simulink model "ClosedLoopSys"  (R2023b)
settings: Solver=VariableStepAuto  StartTime=0.00  StopTime=60.00  FixedStep=T  RelTol=1e-5  EnableMultiTasking=on
values from neighbouring files (symbols this model uses):
  amp_sat_l = 0    [heli_new.m]
  amp_sat_u = 12    [heli_new.m]
  b = fir1(200, 0.004)    [heli_new.m]
  Cr = [1,0,0,0,0,0 ... (first row only)    [heli_new.m]
  DAC_lim_l = 0    [heli_new.m]
  DAC_lim_u = 10    [heli_new.m]
  e_lim_l = min(ElevAxisData.Var1)*pi/180    [heli_new.m]
  Fss_ab = ThrustMeas.Var2    [heli_new.m]
  g = 9.81    [heli_new.m]
  Je = 2*m1*(l1^2)+m2*(l3^2)    (= 0.0023885)    [heli_new.m]
  Jp = 2*m1*(l2^2)    (= 0.0004949)    [heli_new.m]
  Jt = Je    (= 0.0023885)    [heli_new.m]
  K = Kaug(:,1:6)    [heli_new.m]
  k_a = 1.2    [heli_new.m]
  k_d = 0.0005    [heli_new.m]
  k_s = 0.0015    [heli_new.m]
  ki = -Kaug(:,7:8)    [heli_new.m]
  l1 = 0.110    (= 0.11)    [heli_new.m]
  l2 = 0.070    (= 0.07)    [heli_new.m]
  l3 = 0.108    [heli_new.m]
  m1 = 0.0505    [heli_new.m]
  m2 = 0.100    (= 0.1)    [heli_new.m]
  T = 0.02    [heli_new.m]
  tau = 0.6    [heli_new.m]
  U_e = 3.8    [heli_new.m]
  V_ab = ThrustMeas.Var1    [heli_new.m]
undefined symbols (not defined in the file or in its folder): DiscIntNeverNeededParam, kdfilt
settings Model: Creator=bjones  LastModifiedBy=GCRAFT
settings SolverCC: AlgebraicLoopSolver=TrustRegion
settings DataIOCC: SaveFormat=Array  SignalLoggingSaveFormat=ModelDataLogs  ReturnWorkspaceOutputs=off
settings OptimizationCC: BlockReduction=off  BooleanDataType=off  ExpressionDepthLimit=2147483647  LifeSpan=inf
settings DebuggingCC: SaveWithParameterizedLinksMsg=none  UnderspecifiedInitializationDetection=Classic  MergeDetectMultiDrivingBlocksExec=none  SignalResolutionControl=TryResolveAllWithWarning  MultiTaskDSMMsg=warning  MultiTaskCondExecSysMsg=none  FcnCallInpInsideContextMsg=warning  UnconnectedInputMsg=warning  UnconnectedOutputMsg=warning  UnconnectedLineMsg=warning  StateNameClashWarn=warning  SFUnexpectedBacktrackingDiag=warning  SFNoUnconditionalDefaultTransitionDiag=warning  SFExecutionAtInitializationDiag=none  ArithmeticOperatorsInVariantConditions=warning
settings HardwareCC: ProdBitPerPointer=32  ProdBitPerSizeT=32  ProdBitPerPtrDiffT=32  ProdLargestAtomicFloat=None  ProdIntDivRoundTo=Undefined  ProdEndianess=Unspecified  ProdWordSize=32  ProdHWDeviceType=32-bit Generic  TargetUnknown=on
settings ModelReferenceCC: EnableRefExpFcnMdlSchedulingChecks=on  PropagateSignalLabelsOutOfModel=off
settings SFSimCC: SimUseLocalCustomCode=off  CustomCodeUndefinedFunction=UseInterfaceOnly
settings RTWCC: RTWUseLocalCustomCode=off
settings CodeAppCC: StateflowObjectComments=on
settings GRTTargetCC: TargetLangStandard=C89/C90 (ANSI)  CombineOutputUpdateFcns=off  GRTInterface=on
settings ConfigComp: CovMetricSettings=dw  CovSaveCumulativeToWorkspaceVar=on  CovSaveSingleToWorkspaceVar=on  CovExternalEMLEnable=off  CovSFcnEnable=off

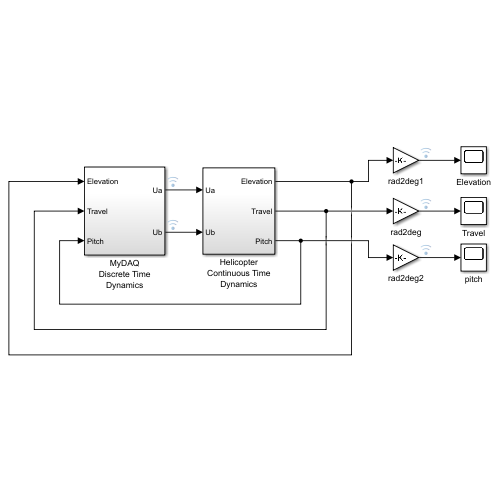
[thumbnail: Simulink's stored preview of the top-level diagram]
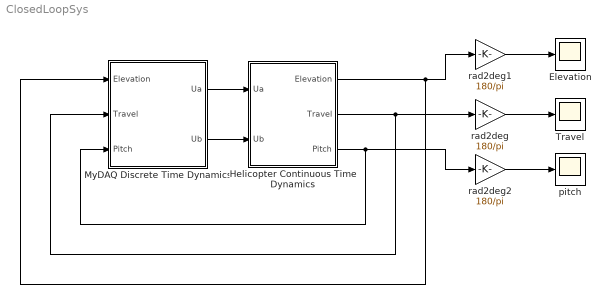
== system ClosedLoopSys ==
  Elevation : Scope
  Helicopter Continuous Time Dynamics : Subsystem
  MyDAQ Discrete Time Dynamics : Subsystem
  Travel : Scope
  pitch : Scope
  rad2deg : Gain  Gain=180/pi  SaturateOnIntegerOverflow=on  OutDataTypeStr=Inherit: Same as input  ParamDataTypeStr=Inherit: Same as input
  rad2deg1 : Gain  Gain=180/pi  SaturateOnIntegerOverflow=on  OutDataTypeStr=Inherit: Same as input  ParamDataTypeStr=Inherit: Same as input
  rad2deg2 : Gain  Gain=180/pi  SaturateOnIntegerOverflow=on  OutDataTypeStr=Inherit: Same as input  ParamDataTypeStr=Inherit: Same as input
  wires:
  rad2deg/1 -> Travel/1
  rad2deg1/1 -> Elevation/1
  Helicopter Continuous Time Dynamics/2(Travel) -> MyDAQ Discrete Time Dynamics/2(Travel), rad2deg/1
  Helicopter Continuous Time Dynamics/1(Elevation) -> rad2deg1/1, MyDAQ Discrete Time Dynamics/1(Elevation)
  rad2deg2/1 -> pitch/1
  Helicopter Continuous Time Dynamics/3(Pitch) -> rad2deg2/1, MyDAQ Discrete Time Dynamics/3(Pitch)
  MyDAQ Discrete Time Dynamics/1(Ua) -> Helicopter Continuous Time Dynamics/1(Ua)
  MyDAQ Discrete Time Dynamics/2(Ub) -> Helicopter Continuous Time Dynamics/2(Ub)

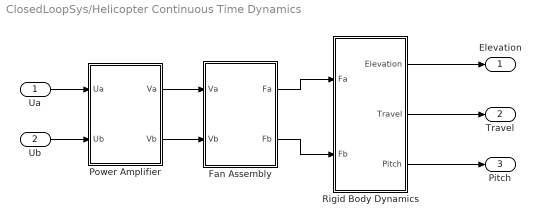
== system ClosedLoopSys/Helicopter Continuous Time Dynamics ==
  Ua : Inport
  Ub : Inport  Port=2
  Fan Assembly : Subsystem
  Power Amplifier : Subsystem
  Rigid Body Dynamics : Subsystem
  Elevation : Outport
  Travel : Outport  Port=2
  Pitch : Outport  Port=3
  wires:
  Power Amplifier/1(Va) -> Fan Assembly/1(Va)
  Power Amplifier/2(Vb) -> Fan Assembly/2(Vb)
  Rigid Body Dynamics/1(Elevation) -> Elevation/1
  Rigid Body Dynamics/3(Pitch) -> Pitch/1
  Fan Assembly/2(Fb) -> Rigid Body Dynamics/2(Fb)
  Ua/1 -> Power Amplifier/1(Ua)
  Ub/1 -> Power Amplifier/2(Ub)
  Rigid Body Dynamics/2(Travel) -> Travel/1
  Fan Assembly/1(Fa) -> Rigid Body Dynamics/1(Fa)

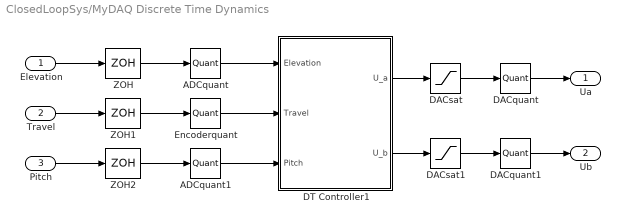
== system ClosedLoopSys/MyDAQ Discrete Time Dynamics ==
  Elevation : Inport
  Travel : Inport  Port=2
  Pitch : Inport  Port=3
  ADCquant : Quantizer  QuantizationInterval=ADC_Vres  SampleTime=T
  ADCquant1 : Quantizer  QuantizationInterval=ADC_Vres  SampleTime=T
  DACquant : Quantizer  QuantizationInterval=DAC_Vres  SampleTime=T
  DACquant1 : Quantizer  QuantizationInterval=DAC_Vres  SampleTime=T
  DACsat : Saturate  UpperLimit=DAC_lim_u  LowerLimit=DAC_lim_l  SampleTime=T
  DACsat1 : Saturate  UpperLimit=DAC_lim_u  LowerLimit=DAC_lim_l  SampleTime=T
  DT Controller1 : Subsystem
  Encoderquant : Quantizer  QuantizationInterval=Encoder_res  SampleTime=T
  ZOH : ZeroOrderHold  SampleTime=T
  ZOH1 : ZeroOrderHold  SampleTime=T
  ZOH2 : ZeroOrderHold  SampleTime=T
  Ua : Outport
  Ub : Outport  Port=2
  wires:
  Elevation/1 -> ZOH/1
  Travel/1 -> ZOH1/1
  DACquant/1 -> Ua/1
  DACquant1/1 -> Ub/1
  DT Controller1/1(U_a) -> DACsat/1
  DACsat/1 -> DACquant/1
  DT Controller1/2(U_b) -> DACsat1/1
  DACsat1/1 -> DACquant1/1
  ZOH1/1 -> Encoderquant/1
  ZOH/1 -> ADCquant/1
  Pitch/1 -> ZOH2/1
  ZOH2/1 -> ADCquant1/1
  ADCquant/1 -> DT Controller1/1(Elevation)
  ADCquant1/1 -> DT Controller1/3(Pitch)
  Encoderquant/1 -> DT Controller1/2(Travel)

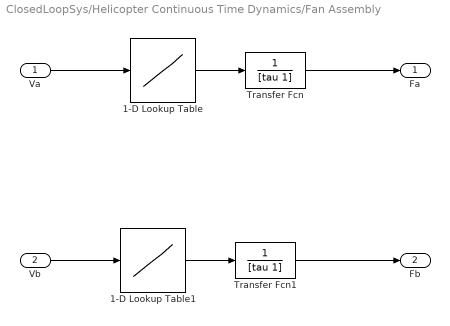
== system ClosedLoopSys/Helicopter Continuous Time Dynamics/Fan Assembly ==
  Va : Inport
  Vb : Inport  Port=2
  1-D Lookup Table : Lookup_n-D  NumberOfTableDimensions=1  LookupTableObject=ThrustMeas  BreakpointsForDimension1=V_ab  Table=Fss_ab  InternalRulePriority=Speed  RndMeth=Simplest
  1-D Lookup Table1 : Lookup_n-D  NumberOfTableDimensions=1  LookupTableObject=ThrustMeas  BreakpointsForDimension1=V_ab  Table=Fss_ab  InternalRulePriority=Speed  RndMeth=Simplest
  Transfer Fcn : TransferFcn  Denominator=[tau 1]
  Transfer Fcn1 : TransferFcn  Denominator=[tau 1]
  Fa : Outport
  Fb : Outport  Port=2
  wires:
  1-D Lookup Table/1 -> Transfer Fcn/1
  Transfer Fcn1/1 -> Fb/1
  1-D Lookup Table1/1 -> Transfer Fcn1/1
  Vb/1 -> 1-D Lookup Table1/1
  Va/1 -> 1-D Lookup Table/1
  Transfer Fcn/1 -> Fa/1

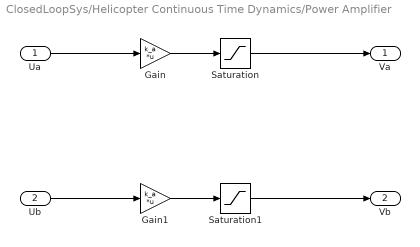
== system ClosedLoopSys/Helicopter Continuous Time Dynamics/Power Amplifier ==
  Ua : Inport
  Ub : Inport  Port=2
  Gain : Gain  Gain=k_a  Multiplication=Matrix(K*u)
  Gain1 : Gain  Gain=k_a  Multiplication=Matrix(K*u)
  Saturation : Saturate  UpperLimit=amp_sat_u  LowerLimit=amp_sat_l
  Saturation1 : Saturate  UpperLimit=amp_sat_u  LowerLimit=amp_sat_l
  Va : Outport
  Vb : Outport  Port=2
  wires:
  Gain/1 -> Saturation/1
  Gain1/1 -> Saturation1/1
  Saturation1/1 -> Vb/1
  Ub/1 -> Gain1/1
  Ua/1 -> Gain/1
  Saturation/1 -> Va/1

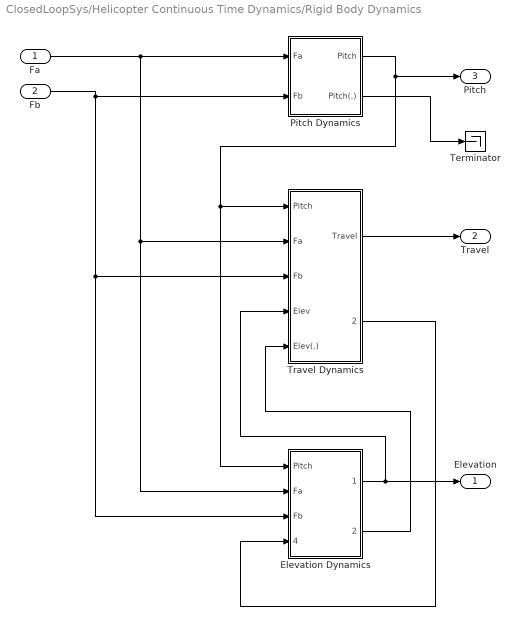
== system ClosedLoopSys/Helicopter Continuous Time Dynamics/Rigid Body Dynamics ==
  Fa : Inport
  Fb : Inport  Port=2
  Elevation Dynamics : Subsystem
  Pitch Dynamics : Subsystem
  Terminator : Terminator
  Travel Dynamics : Subsystem
  Elevation : Outport
  Travel : Outport  Port=2
  Pitch : Outport  Port=3
  wires:
  Fa/1 -> Pitch Dynamics/1(Fa), Travel Dynamics/2(Fa), Elevation Dynamics/2(Fa)
  Fb/1 -> Pitch Dynamics/2(Fb), Elevation Dynamics/3(Fb), Travel Dynamics/3(Fb)
  Travel Dynamics/1(Travel) -> Travel/1
  Elevation Dynamics/1(Elevation) -> Elevation/1, Travel Dynamics/4(Elev)
  Pitch Dynamics/1(Pitch) -> Travel Dynamics/1(Pitch), Elevation Dynamics/1(Pitch), Pitch/1
  Travel Dynamics/2(Travel(.)) -> Elevation Dynamics/4(Travel(.))
  Elevation Dynamics/2(Elevation(.)) -> Travel Dynamics/5(Elev(.))
  Pitch Dynamics/2("Pitch(.) ") -> Terminator/1

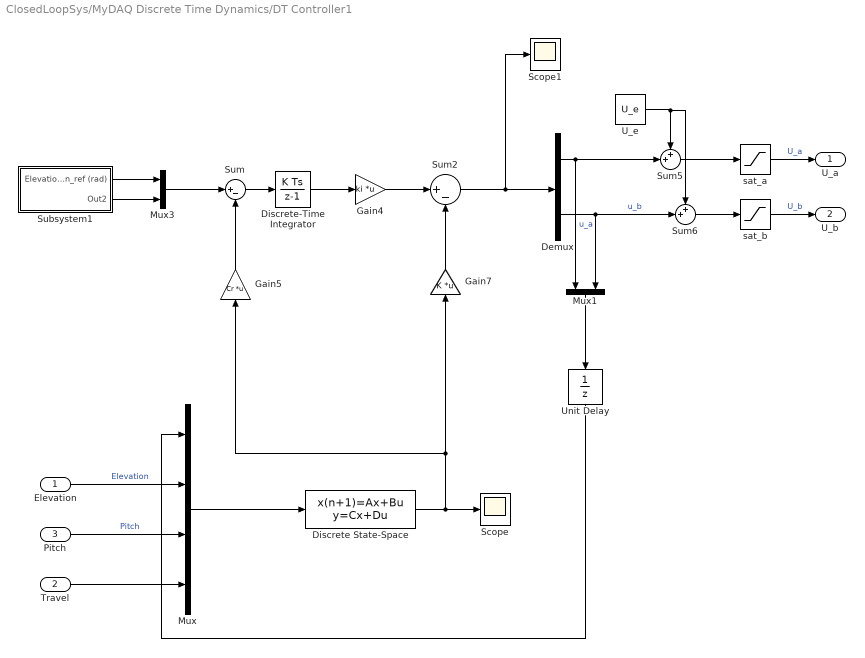
== system ClosedLoopSys/MyDAQ Discrete Time Dynamics/DT Controller1 ==
  Elevation : Inport
  Travel : Inport  Port=2
  Pitch : Inport  Port=3
  Demux : Demux  Outputs=2
  Discrete State-Space : DiscreteStateSpace  A=kdfilt.a  B=kdfilt.b  C=kdfilt.c(size(C,1)+1:end,:)  D=kdfilt.d(size(C,1)+1:end,:)  InitialCondition=[e_lim_l; 0; 0; 0; 0; 0]  SampleTime=T
  Discrete-Time Integrator : DiscreteIntegrator  SampleTime=T  ICPrevOutput=DiscIntNeverNeededParam  ICPrevScaledInput=DiscIntNeverNeededParam
  Gain4 : Gain  Gain=ki  Multiplication=Matrix(K*u)
  Gain5 : Gain  Gain=Cr  Multiplication=Matrix(K*u)
  Gain7 : Gain  Gain=K  Multiplication=Matrix(K*u)
  Mux : Mux
  Mux1 : Mux  Inputs=2
  Mux3 : Mux  Inputs=2
  Scope : Scope
  Scope1 : Scope
  Subsystem1 : Subsystem
  Sum : Sum  Inputs=|+-
  Sum2 : Sum  Inputs=|+-
  Sum5 : Sum  Inputs=++|
  Sum6 : Sum  Inputs=++|
  U_e : Constant  Value=U_e  SampleTime=T
  Unit Delay : UnitDelay  SampleTime=T  HasFrameUpgradeWarning=on
  sat_a : Saturate  UpperLimit=DAC_lim_u  LowerLimit=DAC_lim_l
  sat_b : Saturate  UpperLimit=DAC_lim_u  LowerLimit=DAC_lim_l
  U_a : Outport
  U_b : Outport  Port=2
  wires:
  U_e/1 -> Sum6/1, Sum5/1
  Sum5/1 -> sat_a/1
  Sum6/1 -> sat_b/1
  Demux/1 -> Sum5/2, Mux1/1  "u_a"
  Demux/2 -> Sum6/2, Mux1/2  "u_b"
  Elevation/1 -> Mux/2  "Elevation"
  Discrete-Time Integrator/1 -> Gain4/1
  Sum2/1 -> Scope1/1, Demux/1
  Gain4/1 -> Sum2/1
  Sum/1 -> Discrete-Time Integrator/1
  Pitch/1 -> Mux/3  "Pitch"
  Travel/1 -> Mux/4
  Mux/1 -> Discrete State-Space/1
  Mux1/1 -> Unit Delay/1
  Unit Delay/1 -> Mux/1
  Discrete State-Space/1 -> Scope/1, Gain5/1, Gain7/1
  Mux3/1 -> Sum/1
  Gain5/1 -> Sum/2
  Gain7/1 -> Sum2/2
  Subsystem1/1(Elevation_ref (rad)) -> Mux3/1
  Subsystem1/2(Out2) -> Mux3/2
  sat_a/1 -> U_a/1  "U_a"
  sat_b/1 -> U_b/1  "U_b"

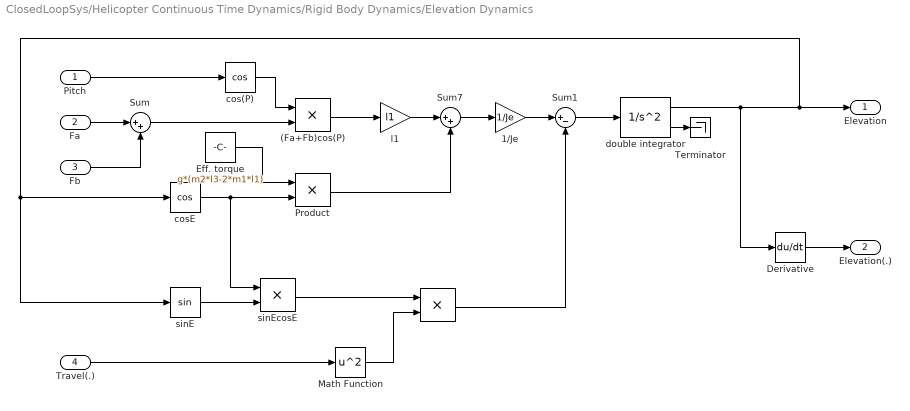
== system ClosedLoopSys/Helicopter Continuous Time Dynamics/Rigid Body Dynamics/Elevation Dynamics ==
  Pitch : Inport
  Fa : Inport  Port=2
  Fb : Inport  Port=3
  Travel(.) : Inport  Port=4
  " " : Product  InputSameDT=on  RndMeth=Zero  SaturateOnIntegerOverflow=on  OutDataTypeStr=Inherit: Same as first input
  (Fa+Fb)cos(P) : Product  InputSameDT=on  RndMeth=Zero  SaturateOnIntegerOverflow=on  OutDataTypeStr=Inherit: Same as first input
  1/Je : Gain  Gain=1/Je  SaturateOnIntegerOverflow=on  OutDataTypeStr=Inherit: Same as input  ParamDataTypeStr=Inherit: Same as input
  Derivative : Derivative
  Eff. torque : Constant  Value=g*(m2*l3-2*m1*l1)
  Math Function : Math  Operator=square  SignedPower=on
  Product : Product  InputSameDT=on  RndMeth=Zero  SaturateOnIntegerOverflow=on  OutDataTypeStr=Inherit: Same as first input
  Sum : Sum  Inputs=|++  InputSameDT=on  SaturateOnIntegerOverflow=on  OutDataTypeStr=Inherit: Same as first input
  Sum1 : Sum  Inputs=|+-  InputSameDT=on  SaturateOnIntegerOverflow=on  OutDataTypeStr=Inherit: Same as first input
  Sum7 : Sum  Inputs=|++  InputSameDT=on  SaturateOnIntegerOverflow=on  OutDataTypeStr=Inherit: Same as first input
  Terminator : Terminator
  cos(P) : Trigonometry  Operator=cos
  cosE : Trigonometry  Operator=cos
  double integrator : SecondOrderIntegrator  ICX=e_lim_l  LimitX=on  UpperLimitX=e_lim_u  LowerLimitX=e_lim_l  LimitDXDT=on  UpperLimitDXDT=2*pi  LowerLimitDXDT=-2*pi
  l1 : Gain  Gain=l1  SaturateOnIntegerOverflow=on  OutDataTypeStr=Inherit: Same as input  ParamDataTypeStr=Inherit: Same as input
  sinE : Trigonometry
  sinEcosE : Product  InputSameDT=on  RndMeth=Zero  SaturateOnIntegerOverflow=on  OutDataTypeStr=Inherit: Same as first input
  Elevation : Outport
  Elevation(.) : Outport  Port=2
  wires:
  double integrator/1 -> cosE/1, sinE/1, Elevation/1, Derivative/1
  Derivative/1 -> Elevation(.)/1
  double integrator/2 -> Terminator/1
  Fa/1 -> Sum/1
  Fb/1 -> Sum/2
  Sum/1 -> (Fa+Fb)cos(P)/2
  Pitch/1 -> cos(P)/1
  cos(P)/1 -> (Fa+Fb)cos(P)/1
  (Fa+Fb)cos(P)/1 -> l1/1
  l1/1 -> Sum7/1
  cosE/1 -> sinEcosE/1, Product/2
  Eff. torque/1 -> Product/1
  sinE/1 -> sinEcosE/2
  Product/1 -> Sum7/2
  Sum7/1 -> 1/Je/1
  1/Je/1 -> Sum1/1
  Travel(.)/1 -> Math Function/1
  Math Function/1 -> " "/2
  sinEcosE/1 -> " "/1
  " "/1 -> Sum1/2
  Sum1/1 -> double integrator/1

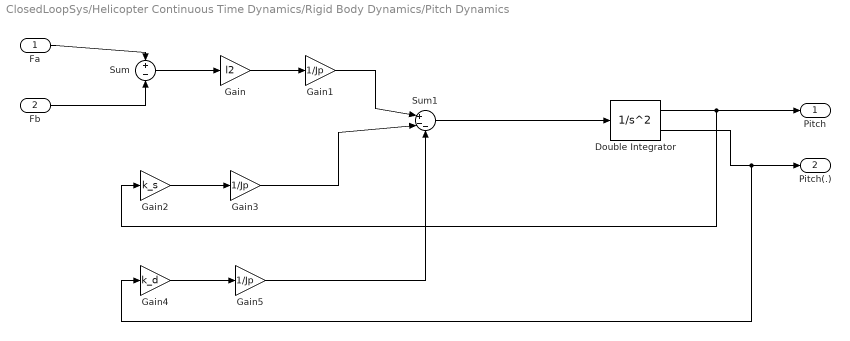
== system ClosedLoopSys/Helicopter Continuous Time Dynamics/Rigid Body Dynamics/Pitch Dynamics ==
  Fa : Inport
  Fb : Inport  Port=2
  Double Integrator : SecondOrderIntegrator  ICX=0  LimitX=on  UpperLimitX=p_lim_u  LowerLimitX=p_lim_l
  Gain : Gain  Gain=l2
  Gain1 : Gain  Gain=1/Jp
  Gain2 : Gain  Gain=k_s
  Gain3 : Gain  Gain=1/Jp
  Gain4 : Gain  Gain=k_d
  Gain5 : Gain  Gain=1/Jp
  Sum : Sum  Inputs=+-
  Sum1 : Sum  Inputs=|+--
  Pitch : Outport
  "Pitch(.) " : Outport  Port=2
  wires:
  Double Integrator/1 -> Gain2/1, Pitch/1
  Fa/1 -> Sum/1
  Fb/1 -> Sum/2
  Sum/1 -> Gain/1
  Gain/1 -> Gain1/1
  Gain1/1 -> Sum1/1
  Gain2/1 -> Gain3/1
  Gain3/1 -> Sum1/2
  Gain4/1 -> Gain5/1
  Gain5/1 -> Sum1/3
  Sum1/1 -> Double Integrator/1
  Double Integrator/2 -> Gain4/1, "Pitch(.) "/1

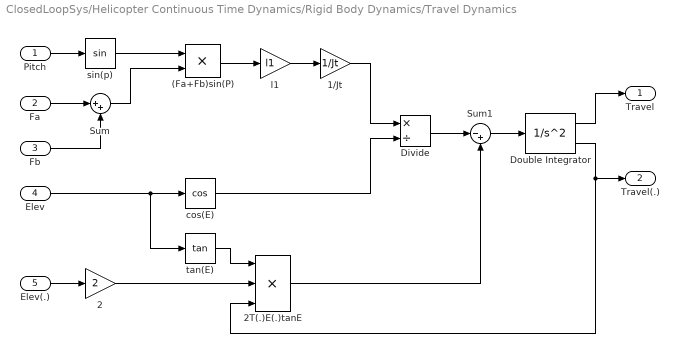
== system ClosedLoopSys/Helicopter Continuous Time Dynamics/Rigid Body Dynamics/Travel Dynamics ==
  Pitch : Inport
  Fa : Inport  Port=2
  Fb : Inport  Port=3
  Elev : Inport  Port=4
  Elev(.) : Inport  Port=5
  (Fa+Fb)sin(P) : Product  InputSameDT=on  RndMeth=Zero  SaturateOnIntegerOverflow=on  OutDataTypeStr=Inherit: Same as first input
  1/Jt : Gain  Gain=1/Jt  SaturateOnIntegerOverflow=on  OutDataTypeStr=Inherit: Same as input  ParamDataTypeStr=Inherit: Same as input
  2 : Gain  Gain=2  SaturateOnIntegerOverflow=on  OutDataTypeStr=Inherit: Same as input  ParamDataTypeStr=Inherit: Same as input
  2T(.)E(.)tanE : Product  Inputs=3  InputSameDT=on  RndMeth=Zero  SaturateOnIntegerOverflow=on  OutDataTypeStr=Inherit: Same as first input
  Divide : Product  Inputs=*/
  Double Integrator : SecondOrderIntegrator  UpperLimitX=1  LowerLimitX=0  LimitDXDT=on  UpperLimitDXDT=2  LowerLimitDXDT=-2
  Sum : Sum  Inputs=|++  InputSameDT=on  SaturateOnIntegerOverflow=on  OutDataTypeStr=Inherit: Same as first input
  Sum1 : Sum  Inputs=|-+  InputSameDT=on  SaturateOnIntegerOverflow=on  OutDataTypeStr=Inherit: Same as first input
  cos(E) : Trigonometry  Operator=cos
  l1 : Gain  Gain=l1  SaturateOnIntegerOverflow=on  OutDataTypeStr=Inherit: Same as input  ParamDataTypeStr=Inherit: Same as input
  sin(p) : Trigonometry
  tan(E) : Trigonometry  Operator=tan
  Travel : Outport
  Travel(.) : Outport  Port=2
  wires:
  Double Integrator/1 -> Travel/1
  sin(p)/1 -> (Fa+Fb)sin(P)/1
  (Fa+Fb)sin(P)/1 -> l1/1
  Pitch/1 -> sin(p)/1
  Fa/1 -> Sum/1
  Fb/1 -> Sum/2
  Sum/1 -> (Fa+Fb)sin(P)/2
  l1/1 -> 1/Jt/1
  Elev/1 -> cos(E)/1, tan(E)/1
  1/Jt/1 -> Divide/1
  cos(E)/1 -> Divide/2
  Double Integrator/2 -> Travel(.)/1, 2T(.)E(.)tanE/3
  tan(E)/1 -> 2T(.)E(.)tanE/1
  Elev(.)/1 -> 2/1
  2/1 -> 2T(.)E(.)tanE/2
  Divide/1 -> Sum1/1
  Sum1/1 -> Double Integrator/1
  2T(.)E(.)tanE/1 -> Sum1/2

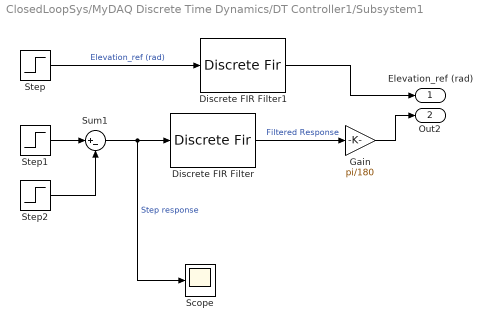
== system ClosedLoopSys/MyDAQ Discrete Time Dynamics/DT Controller1/Subsystem1 ==
  Discrete FIR Filter : DiscreteFir  Coefficients=b  InputProcessing=Columns as channels (frame based)
  Discrete FIR Filter1 : DiscreteFir  Coefficients=b  InputProcessing=Columns as channels (frame based)
  Gain : Gain  Gain=pi/180
  Scope : Scope
  Step : Step  Time=0  Before=e_lim_l  After=0  SampleTime=T
  Step1 : Step  Time=20  After=180  SampleTime=T
  Step2 : Step  Time=40  After=180  SampleTime=T
  Sum1 : Sum  Inputs=|+-
  Elevation_ref (rad) : Outport
  Out2 : Outport  Port=2
  wires:
  Gain/1 -> Out2/1
  Sum1/1 -> Discrete FIR Filter/1, Scope/1  "Step response"
  Step1/1 -> Sum1/1
  Step2/1 -> Sum1/2
  Discrete FIR Filter/1 -> Gain/1  "Filtered Response"
  Step/1 -> Discrete FIR Filter1/1  "Elevation_ref (rad)"
  Discrete FIR Filter1/1 -> Elevation_ref (rad)/1
